simulink model "FM_system"  (R2021a)
settings: Solver=VariableStepAuto  StartTime=0.0  StopTime=10.0  RelTol=1e-3
settings Model: Creator=Fatiha  LastModifiedBy=Fatiha

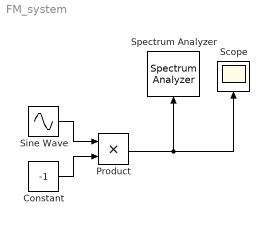
== system FM_system ==
  Constant : Constant  Value=-1
  Product : Product
  Scope : Scope
  Sine Wave : Sin  Frequency=2*pi*50  SampleTime=0.0001
  Spectrum Analyzer : SpectrumAnalyzer
  wires:
  Sine Wave/1 -> Product/1
  Constant/1 -> Product/2
  Product/1 -> Scope/1, Spectrum Analyzer/1
